simulink subsystem "Subsystem_Plant_BAv03"  (R2023a)
settings: Solver=VariableStepAuto  StartTime=0.0  StopTime=10.0  RelTol=1e-3
undefined symbols (not defined in the file): driver, param, route
libraries: simulink x1
settings Model: Creator=giaco  LastModifiedBy=giaco
settings OptimizationCC: ReuseModelBlockBuffer=off

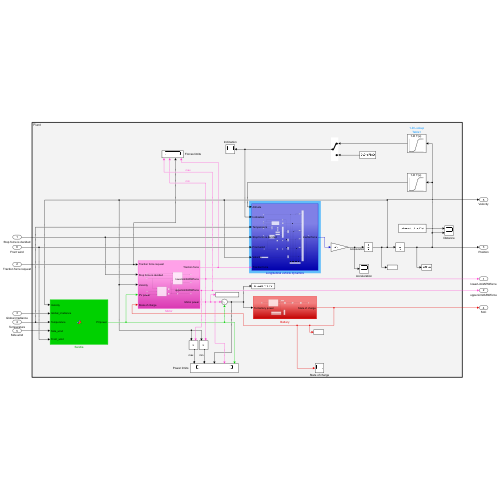
[thumbnail: Simulink's stored preview of the top-level diagram]
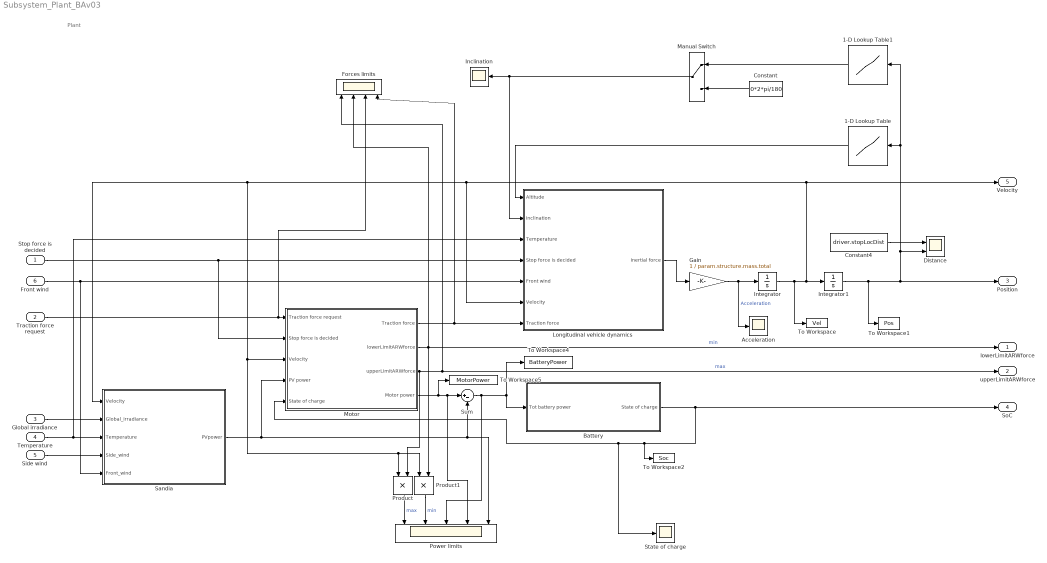
== system Subsystem_Plant_BAv03 ==
  note: Plant
  Stop force is decided : Inport  OutDataTypeStr=boolean
  Traction force request : Inport  Port=2
  Global irradiance : Inport  Port=3
  Temperature : Inport  Port=4
  Side wind : Inport  Port=5
  Front wind : Inport  Port=6
  1-D Lookup Table : Lookup_n-D  NumberOfTableDimensions=1  BreakpointsForDimension1=route.dist  Table=route.altiSmooth  InternalRulePriority=Speed  RndMeth=Simplest
  1-D Lookup Table1 : Lookup_n-D  NumberOfTableDimensions=1  BreakpointsForDimension1=route.dist(1:end-1)  Table=route.inclSmooth  InternalRulePriority=Speed  RndMeth=Simplest
  Acceleration : Scope
  Battery : Subsystem
  Constant : Constant  Value=0*2*pi/180
  Constant4 : Constant  Value=driver.stopLocDist
  Distance : Scope  NumInputPorts=2
  Forces limits : Scope  NumInputPorts=4
  Gain : Gain  Gain=1 / param.structure.mass.total
  Inclination : Scope
  Integrator : Integrator
  Integrator1 : Integrator
  Longitudinal vehicle dynamics : Subsystem
  Manual Switch : ManualSwitch
  Motor : Subsystem
  Power limits : Scope  NumInputPorts=5
  Product : Product
  Product1 : Product
  Sandia : MATLAB Function  TreatAsAtomicUnit=on
  State of charge : Scope
  Sum : Sum  Inputs=|+-
  To Workspace : ToWorkspace  VariableName=Vel  SaveFormat=Timeseries  SampleTime=-1
  To Workspace1 : ToWorkspace  VariableName=Pos  SaveFormat=Timeseries  SampleTime=-1
  To Workspace2 : ToWorkspace  VariableName=Soc  SaveFormat=Timeseries  SampleTime=-1
  To Workspace4 : ToWorkspace  VariableName=BatteryPower  SaveFormat=Timeseries  SampleTime=-1
  To Workspace5 : ToWorkspace  VariableName=MotorPower  SaveFormat=Timeseries  SampleTime=-1
  lowerLimitARWforce : Outport
  upperLimitARWforce : Outport  Port=2
  Position : Outport  Port=3
  SoC : Outport  Port=4
  Velocity : Outport  Port=5
  wires:
  Integrator/1 -> To Workspace/1, Velocity/1, Longitudinal vehicle dynamics/6(Velocity), Product/1, Product1/1, Motor/3(Velocity), Sandia/1(Velocity), Integrator1/1
  Battery/1(State of charge) -> SoC/1, To Workspace2/1, Motor/5(State of charge), State of charge/1
  Longitudinal vehicle dynamics/1(Inertial force) -> Gain/1
  Manual Switch/1 -> Inclination/1, Longitudinal vehicle dynamics/2(Inclination)
  Traction force request/1 -> Motor/1(Traction force request), Forces limits/3
  Gain/1 -> Integrator/1, Acceleration/1  "Acceleration"
  Sum/1 -> Power limits/3, Battery/1(Tot battery power), To Workspace4/1
  Integrator1/1 -> To Workspace1/1, 1-D Lookup Table/1, 1-D Lookup Table1/1, Distance/2, Position/1
  Sandia/1(PVpower) -> Sum/2, Power limits/5, Motor/4(PV power)
  Motor/4(Motor power) -> To Workspace5/1, Power limits/4, Sum/1
  Stop force is decided/1 -> Motor/2(Stop force is decided), Longitudinal vehicle dynamics/4(Stop force is decided)
  Constant/1 -> Manual Switch/2
  Motor/1(Traction force) -> Longitudinal vehicle dynamics/7(Traction force), Forces limits/4
  Global irradiance/1 -> Sandia/2(Global_irradiance)
  Temperature/1 -> Longitudinal vehicle dynamics/3(Temperature), Sandia/3(Temperature)
  Side wind/1 -> Sandia/4(Side_wind)
  Front wind/1 -> Sandia/5(Front_wind), Longitudinal vehicle dynamics/5(Front wind)
  Product/1 -> Power limits/1  "max"
  Product1/1 -> Power limits/2  "min"
  Motor/3(upperLimitARWforce) -> Product/2, upperLimitARWforce/1, Forces limits/1  "max"
  Motor/2(lowerLimitARWforce) -> lowerLimitARWforce/1, Forces limits/2, Product1/2  "min"
  Constant4/1 -> Distance/1
  1-D Lookup Table1/1 -> Manual Switch/1
  1-D Lookup Table/1 -> Longitudinal vehicle dynamics/1(Altitude)

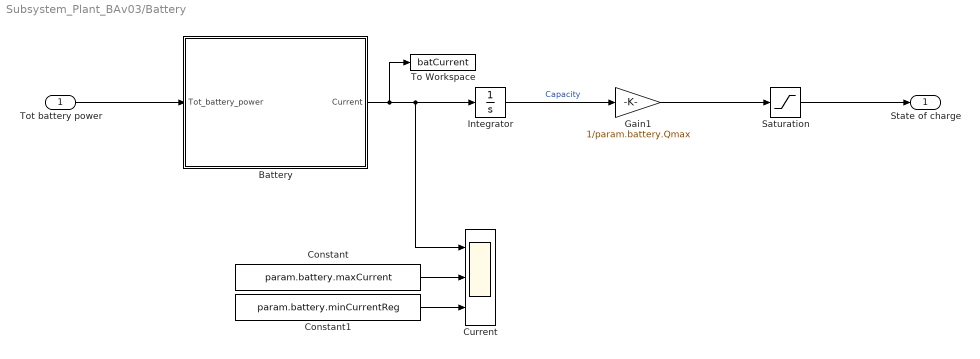
== system Subsystem_Plant_BAv03/Battery ==
  Tot battery power : Inport
  Battery : MATLAB Function  TreatAsAtomicUnit=on
  Constant : Constant  Value=param.battery.maxCurrent
  Constant1 : Constant  Value=param.battery.minCurrentReg
  Current : Scope  NumInputPorts=3
  Gain1 : Gain  Gain=1/param.battery.Qmax
  Integrator : Integrator  InitialCondition=param.battery.Qmax
  Saturation : Saturate  UpperLimit=1  LowerLimit=-Inf
  To Workspace : ToWorkspace  VariableName=batCurrent  SaveFormat=Timeseries  SampleTime=-1
  State of charge : Outport
  wires:
  Constant1/1 -> Current/3
  Constant/1 -> Current/2
  Battery/1(Current) -> Integrator/1, Current/1, To Workspace/1
  Integrator/1 -> Gain1/1  "Capacity"
  Gain1/1 -> Saturation/1
  Tot battery power/1 -> Battery/1(Tot_battery_power)
  Saturation/1 -> State of charge/1

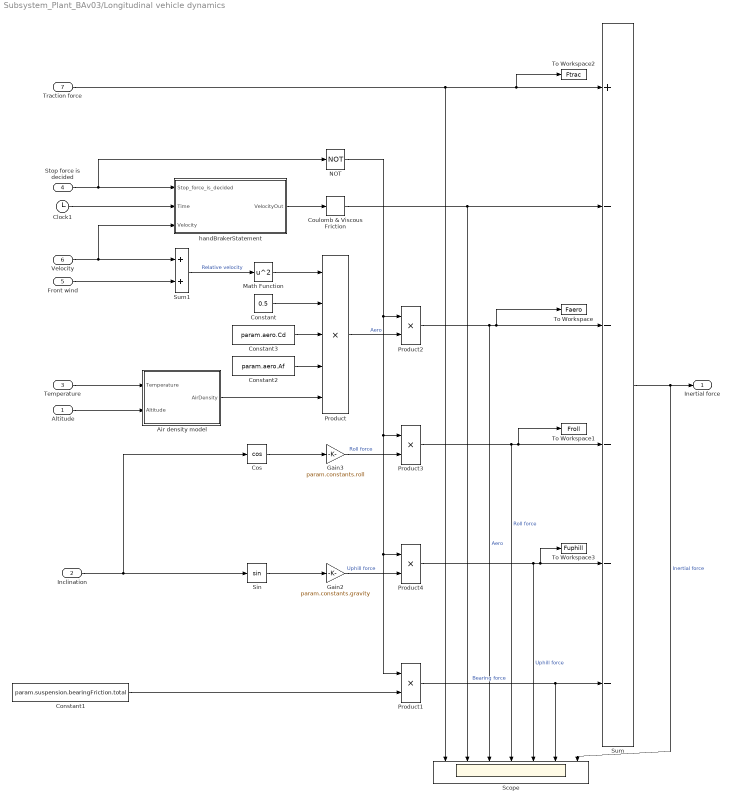
== system Subsystem_Plant_BAv03/Longitudinal vehicle dynamics ==
  Altitude : Inport
  Inclination : Inport  Port=2
  Temperature : Inport  Port=3
  Stop force is decided : Inport  Port=4
  Front wind : Inport  Port=5
  Velocity : Inport  Port=6
  Traction force : Inport  Port=7
  Air density model : MATLAB Function  TreatAsAtomicUnit=on
  Clock1 : Clock
  Constant : Constant  Value=0.5
  Constant1 : Constant  Value=param.suspension.bearingFriction.total
  Constant2 : Constant  Value=param.aero.Af
  Constant3 : Constant  Value=param.aero.Cd
  Cos : Trigonometry  Operator=cos
  Coulomb & Viscous Friction : simulink/Discontinuities/Coulomb & Viscous Friction  offset=0  gain=1000
  Gain2 : Gain  Gain=param.constants.gravity
  Gain3 : Gain  Gain=param.constants.roll
  Math Function : Math  Operator=square
  NOT : Logic  Operator=NOT  IconShape=distinctive  AllPortsSameDT=off  OutDataTypeStr=boolean
  Product : Product  Inputs=5
  Product{1..4} (4 alike) : Product
  Scope : Scope  NumInputPorts=7
  Sin : Trigonometry
  Sum : Sum  Inputs=+-----
  Sum1 : Sum
  To Workspace : ToWorkspace  VariableName=Faero  SaveFormat=Timeseries  SampleTime=-1
  To Workspace1 : ToWorkspace  VariableName=Froll  SaveFormat=Timeseries  SampleTime=-1
  To Workspace2 : ToWorkspace  VariableName=Ftrac  SaveFormat=Timeseries  SampleTime=-1
  To Workspace3 : ToWorkspace  VariableName=Fuphill  SaveFormat=Timeseries  SampleTime=-1
  handBrakerStatement : MATLAB Function  TreatAsAtomicUnit=on
  Inertial force : Outport
  wires:
  Constant1/1 -> Product1/2
  Product1/1 -> Sum/6, Scope/6  "Bearing force"
  Traction force/1 -> To Workspace2/1, Sum/1, Scope/1
  Gain2/1 -> Product4/2  "Uphill force"
  Gain3/1 -> Product3/2  "Roll force"
  NOT/1 -> Product4/1, Product1/1, Product3/1, Product2/1
  Product/1 -> Product2/2  "Aero"
  Clock1/1 -> handBrakerStatement/2(Time)
  handBrakerStatement/1(VelocityOut) -> Coulomb & Viscous Friction/1
  Coulomb & Viscous Friction/1 -> Sum/2, Scope/2
  Stop force is decided/1 -> NOT/1, handBrakerStatement/1(Stop_force_is_decided)
  Product2/1 -> To Workspace/1, Sum/3, Scope/3  "Aero"
  Product3/1 -> To Workspace1/1, Sum/4, Scope/4  "Roll force"
  Cos/1 -> Gain3/1
  Math Function/1 -> Product/1
  Inclination/1 -> Sin/1, Cos/1
  Sin/1 -> Gain2/1
  Product4/1 -> To Workspace3/1, Sum/5, Scope/5  "Uphill force"
  Velocity/1 -> handBrakerStatement/3(Velocity), Sum1/1
  Sum/1 -> Inertial force/1, Scope/7  "Inertial force"
  Front wind/1 -> Sum1/2
  Sum1/1 -> Math Function/1  "Relative velocity"
  Temperature/1 -> Air density model/1(Temperature)
  Altitude/1 -> Air density model/2(Altitude)
  Air density model/1(AirDensity) -> Product/5
  Constant2/1 -> Product/4
  Constant3/1 -> Product/3
  Constant/1 -> Product/2

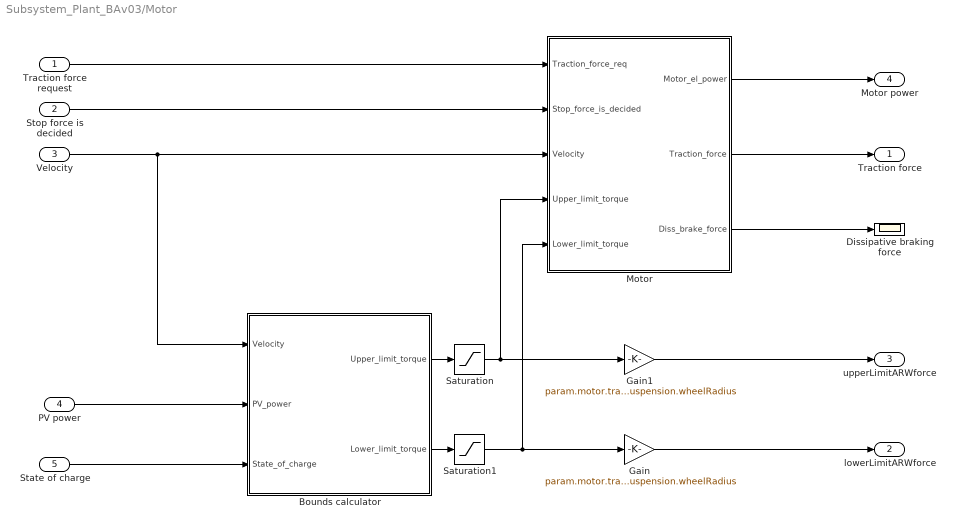
== system Subsystem_Plant_BAv03/Motor ==
  Traction force request : Inport
  Stop force is decided : Inport  Port=2
  Velocity : Inport  Port=3
  PV power : Inport  Port=4
  State of charge : Inport  Port=5
  Bounds calculator : MATLAB Function  TreatAsAtomicUnit=on
  Dissipative braking force : Scope
  Gain : Gain  Gain=param.motor.transmissionRatio / param.suspension.wheelRadius
  Gain1 : Gain  Gain=param.motor.transmissionRatio / param.suspension.wheelRadius
  Motor : MATLAB Function  TreatAsAtomicUnit=on
  Saturation : Saturate  UpperLimit=Inf  LowerLimit=0
  Saturation1 : Saturate  UpperLimit=0  LowerLimit=-Inf
  Traction force : Outport
  lowerLimitARWforce : Outport  Port=2
  upperLimitARWforce : Outport  Port=3
  Motor power : Outport  Port=4
  wires:
  Saturation1/1 -> Gain/1, Motor/5(Lower_limit_torque)
  Saturation/1 -> Gain1/1, Motor/4(Upper_limit_torque)
  Bounds calculator/1(Upper_limit_torque) -> Saturation/1
  Bounds calculator/2(Lower_limit_torque) -> Saturation1/1
  State of charge/1 -> Bounds calculator/3(State_of_charge)
  Traction force request/1 -> Motor/1(Traction_force_req)
  Velocity/1 -> Motor/3(Velocity), Bounds calculator/1(Velocity)
  Motor/1(Motor_el_power) -> Motor power/1
  Motor/2(Traction_force) -> Traction force/1
  Motor/3(Diss_brake_force) -> Dissipative braking force/1
  PV power/1 -> Bounds calculator/2(PV_power)
  Stop force is decided/1 -> Motor/2(Stop_force_is_decided)
  Gain1/1 -> upperLimitARWforce/1
  Gain/1 -> lowerLimitARWforce/1

== matlab function Subsystem_Plant_BAv03/Battery/Battery ==
  data: Tot_battery_power input; Current output; param parameter
function Current = fcn(Tot_battery_power, param)

%conversion to single battery power
Battery_power = Tot_battery_power ./ param.battery.totNum;

%solution of quadratic equation
Current_befEff = (param.battery.Uoc - sqrt(param.battery.Uoc^2 - 4*Battery_power*param.battery.R)) / (2*param.battery.R);

%Coulomb efficiency
Current = - param.battery.effCoul .* Current_befEff;

== matlab function Subsystem_Plant_BAv03/Longitudinal vehicle dynamics/Air density model ==
  data: Temperature input; AirDensity output; Altitude input; param parameter
function AirDensity = fcn(Temperature, Altitude, param)

Temp_K = Temperature + 273.15;

AirDensity = param.air.p0 * param.air.M ./ (param.air.R * Temp_K) .* exp(-param.air.M * param.constants.g * Altitude ./ (param.air.R * Temp_K));
end % fct

== matlab function Subsystem_Plant_BAv03/Sandia ==
  data: Velocity input; Global_irradiance input; Temperature input; PVpower output; Side_wind input; Front_wind input; param parameter
function PVpower = fcn(Velocity, Global_irradiance, Temperature, Side_wind, Front_wind, param)

type = 2;
mounting = 1;

relVelocity = Velocity + Front_wind;
effVelocity = sqrt(relVelocity^2 + Side_wind^2);

tempCell = cellTemperatureSandiaSim(Global_irradiance, Temperature, effVelocity, type, mounting);

PVpower = param.pv.area * Global_irradiance * param.pv.eff * (1 + param.pv.powerCoeff * (tempCell - param.pv.tempSTC)) * param.pv.loss.total;

== matlab function Subsystem_Plant_BAv03/Motor/Bounds calculator ==
  data: Velocity input; PV_power input; State_of_charge input; param parameter; Upper_limit_torque output; Lower_limit_torque output
function [Upper_limit_torque, Lower_limit_torque] = boundsCalculator(Velocity, PV_power, State_of_charge, param)

%%  Conversion battery limits
minElPowerMotBat = param.battery.lowerBoundPower * param.battery.totNum + PV_power;
minMechPowerMotBat = elPower2mechPower_Willans(minElPowerMotBat, param);

maxElPowerMotBat = param.battery.upperBoundPower * param.battery.totNum + PV_power;
maxMechPowerMotBat = elPower2mechPower_Willans(maxElPowerMotBat, param);

%state of charge relation
SoCwendePunkt = 0.10; %-
if State_of_charge < SoCwendePunkt
    maxPowerSoC = maxMechPowerMotBat / SoCwendePunkt * State_of_charge;
else
    maxPowerSoC = maxMechPowerMotBat;
end % if

%% Torque and rotational speed
omegaMot = Velocity * param.motor.transmissionRatio/param.suspension.wheelRadius;

%% Lower limit
Lower_limit_torque = max(param.motor.minTorque, param.motor.minPower / max(omegaMot, 1e-8)); %lower limit power motor
Lower_limit_torque = max(Lower_limit_torque, minMechPowerMotBat / max(omegaMot, 1e-8)); %lower limit power battery

%% Upper limit
Upper_limit_torque = min(param.motor.maxTorque, param.motor.maxPower / max(omegaMot, 1e-8)); %upper limit power motor
Upper_limit_torque = min(Upper_limit_torque, maxMechPowerMotBat / max(omegaMot, 1e-8)); %upper limit power battery
Upper_limit_torque = min(Upper_limit_torque, maxPowerSoC / max(omegaMot, 1e-8)); %upper limit state of charge

end % fct

== matlab function Subsystem_Plant_BAv03/Motor/Motor ==
  data: Traction_force_req input; Stop_force_is_decided input; Velocity input; Upper_limit_torque input; Lower_limit_torque input; param parameter; Motor_el_power output; Traction_force output; Diss_brake_force output
function [Motor_el_power, Traction_force, Diss_brake_force] = Motor(Traction_force_req, Stop_force_is_decided, Velocity, Upper_limit_torque, Lower_limit_torque, param)

Diss_brake_force = 0;

%% Standing condition
if Stop_force_is_decided
    Traction_force = 0;
    Motor_el_power = 0;

else
%% Conversions
    tractionTorqueReq = Traction_force_req * param.suspension.wheelRadius/param.motor.transmissionRatio;
    omegaMot = Velocity * param.motor.transmissionRatio/param.suspension.wheelRadius;

%% Limits
    tractionTorque = tractionTorqueReq;
    tractionTorque = min(tractionTorque, Upper_limit_torque); %upper limit
    tractionTorque = max(tractionTorque, Lower_limit_torque); %lower limit
    
%% Electric motor power
    mechPower = omegaMot * tractionTorque;
    Motor_el_power = mechPower2elPower_Willans(mechPower, param);

%% Traction force
    Traction_force = tractionTorque * param.motor.transmissionRatio / param.suspension.wheelRadius;

    %additional dissipative braking force
    deltaBrake = Traction_force_req - Traction_force;
    if deltaBrake < 0
        Diss_brake_force = deltaBrake;
        Traction_force = Traction_force + Diss_brake_force;
    end % if
end % if
end % fct

== matlab function Subsystem_Plant_BAv03/Longitudinal vehicle dynamics/handBrakerStatement ==
  data: Stop_force_is_decided input; Time input; Velocity input; VelocityOut output
function VelocityOut = handBrakerStatement(Stop_force_is_decided, Time, Velocity)

VelocityOut = 0;

if Stop_force_is_decided || (Velocity < 0 && Time > 10)
    VelocityOut = Velocity;
end % if
